simulink library "DAMA_lib"  (Simulink 6.6)
undefined symbols (not defined in the file or in its folder): aa2rot, D, DiscIntNeverNeededParam, DRprogressbar, epsilon, Kd, Ko, Kp, manip, manipulator, path_des, Q, q0, q_d0, rho, robot, show_3D, StartTime, subs, Ts, VR_handle, vrmfunc
libraries: DAMA_lib x7, vrlib x1, simulink x1
(part 2 of 4)

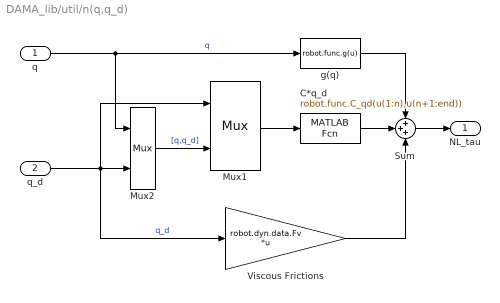
== system DAMA_lib/util/n(q,q_d) ==
  q : Inport
  q_d : Inport  Port=2
  C*q_d : MATLABFcn  MATLABFcn=robot.func.C_qd(u(1:n),u(n+1:end))  OutputDimensions=n
  Mux1 : Mux  Inputs=2
      settings: DisplayOption=signals
  Mux2 : Mux  Inputs=2
      settings: DisplayOption=signals
  Sum : Sum  Inputs=+++
  Viscous Frictions : Gain  Gain=robot.dyn.data.Fv  Multiplication=Matrix(K*u)
  g(q) : MATLABFcn  MATLABFcn=robot.func.g(u)  OutputDimensions=n
  NL_tau : Outport
  wires:
  Viscous Frictions/1 -> Sum/3
  Sum/1 -> NL_tau/1
  q/1 -> g(q)/1, Mux2/1  "q"
  q_d/1 -> Viscous Frictions/1, Mux1/1, Mux2/2  "q_d"
  C*q_d/1 -> Sum/2
  g(q)/1 -> Sum/1
  Mux2/1 -> Mux1/2  "[q,q_d]"
  Mux1/1 -> C*q_d/1

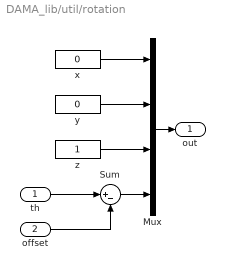
== system DAMA_lib/util/rotation ==
  th : Inport
  offset : Inport  Port=2
  Mux : Mux
  Sum : Sum  Inputs=|+-
  x : Constant  Value=0
  y : Constant  Value=0
  z : Constant
  out : Outport
  wires:
  offset/1 -> Sum/2
  Sum/1 -> Mux/4
  th/1 -> Sum/1
  Mux/1 -> out/1
  z/1 -> Mux/3
  y/1 -> Mux/2
  x/1 -> Mux/1

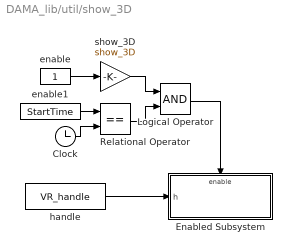
== system DAMA_lib/util/show_3D ==
  Clock : Clock
      settings: Decimation=10
  Enabled Subsystem : Subsystem  TreatAsAtomicUnit=on
  Logical Operator : Logic  AllPortsSameDT=off  OutDataTypeMode=Boolean
  Relational Operator : RelationalOperator  Operator===  LogicOutDataTypeMode=Boolean
  enable : Constant
  enable1 : Constant  Value=StartTime
  handle : Constant  Value=VR_handle
  show_3D : Gain  Gain=show_3D
  wires:
  show_3D/1 -> Logical Operator/1
  enable/1 -> show_3D/1
  handle/1 -> Enabled Subsystem/1(h)
  Logical Operator/1 -> Enabled Subsystem/Enable
  Relational Operator/1 -> Logical Operator/2
  enable1/1 -> Relational Operator/1
  Clock/1 -> Relational Operator/2

== system DAMA_lib/util/translation ==
  d : Inport
  offset : Inport  Port=2
  Mux : Mux  Inputs=3
  Sum : Sum  Inputs=|+-
  x : Constant  Value=0
  y : Constant  Value=0
  out : Outport
  wires:
  offset/1 -> Sum/2
  Sum/1 -> Mux/3
  d/1 -> Sum/1
  Mux/1 -> out/1
  y/1 -> Mux/2
  x/1 -> Mux/1

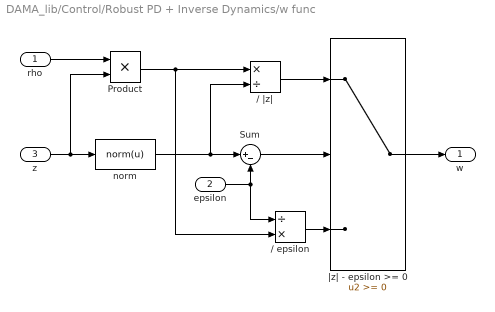
== system DAMA_lib/Control/Robust PD + Inverse Dynamics/w func ==
  rho : Inport
  epsilon : Inport  Port=2
  z : Inport  Port=3
  " / epsilon" : Product  Inputs=/*  OutScaling=2^-10
  " / |z|" : Product  Inputs=*/  OutScaling=2^-10
  Product : Product  RndMeth=Zero
  Sum : Sum  Inputs=|+-
  norm : MATLABFcn  MATLABFcn=norm(u)
  |z| - epsilon >= 0 : Switch
  w : Outport
  wires:
  z/1 -> norm/1, Product/2
  Sum/1 -> |z| - epsilon >= 0/2
  rho/1 -> Product/1
  norm/1 -> Sum/1, " / |z|"/2
  Product/1 -> " / |z|"/1, " / epsilon"/2
  " / |z|"/1 -> |z| - epsilon >= 0/1
  " / epsilon"/1 -> |z| - epsilon >= 0/3
  epsilon/1 -> Sum/2, " / epsilon"/1
  |z| - epsilon >= 0/1 -> w/1

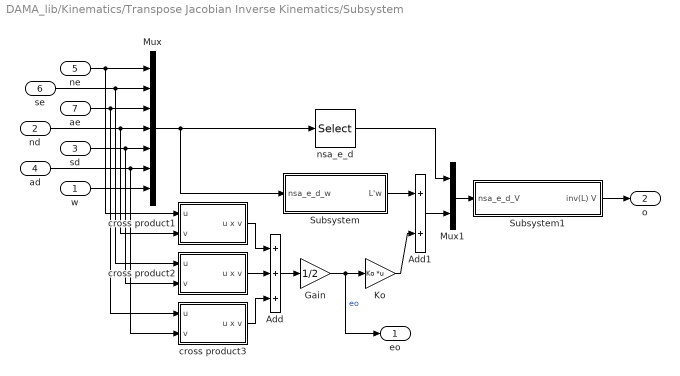
== system DAMA_lib/Kinematics/Transpose Jacobian Inverse Kinematics/Subsystem ==
  w : Inport
  nd : Inport  Port=2
  sd : Inport  Port=3
  ad : Inport  Port=4
  ne : Inport  Port=5
  se : Inport  Port=6
  ae : Inport  Port=7
  Add : Sum  Inputs=3  OutScaling=2^-10
  Add1 : Sum  Inputs=2  OutScaling=2^-10
  Gain : Gain  Gain=1/2
  Ko : Gain  Gain=Ko  Multiplication=Matrix(K*u) (u vector)
  Mux : Mux  Inputs=7
  Mux1 : Mux  Inputs=2
  Subsystem : Subsystem
  Subsystem1 : Subsystem
  cross product1 : Subsystem
  cross product2 : Subsystem
  cross product3 : Subsystem
  nsa_e_d : Selector  IndexOptions=Index vector (dialog)  Indices=[1:18]  OutputSizes=1  InputPortWidth=21
  eo : Outport
  o : Outport  Port=2
  wires:
  ne/1 -> Mux/1, cross product1/1(u)
  se/1 -> Mux/2, cross product2/1(u)
  ae/1 -> Mux/3, cross product3/1(u)
  nd/1 -> Mux/4, cross product1/2(v)
  sd/1 -> Mux/5, cross product2/2(v)
  ad/1 -> Mux/6, cross product3/2(v)
  w/1 -> Mux/7
  cross product1/1(u x v) -> Add/1
  cross product2/1(u x v) -> Add/2
  cross product3/1(u x v) -> Add/3
  Add/1 -> Gain/1
  Gain/1 -> eo/1, Ko/1  "eo"
  nsa_e_d/1 -> Mux1/1
  Mux1/1 -> Subsystem1/1(nsa_e_d_V)
  Mux/1 -> Subsystem/1(nsa_e_d_w), nsa_e_d/1
  Subsystem/1(L'w) -> Add1/1
  Ko/1 -> Add1/2
  Add1/1 -> Mux1/2
  Subsystem1/1(inv(L) V) -> o/1

== system DAMA_lib/util/show_3D/Enabled Subsystem ==
  h : Inport
  Enable : EnablePort
  show 3D : MATLABFcn  MATLABFcn=vrmfunc('FnOpen', u )  OutputDimensions=0
  wires:
  h/1 -> show 3D/1

== system DAMA_lib/Kinematics/Transpose Jacobian Inverse Kinematics/Subsystem/Subsystem ==
  nsa_e_d_w : Inport
  L'1 : Fcn  Expr=(1/2*u(12)*u(3)+1/2*u(11)*u(2)+1/2*u(15)*u(6)+1/2*u(14)*u(5)+1/2*u(18)*u(9)+1/2*u(17)*u(8))*u(19)+(-1/2*u(10)*u(2)-1/2*u(13)*u(5)-1/2*u(16)*u(8))*u(20)+(-1/2*u(10)*u(3)-1/2*u(13)*u(6)-1/2*u(16)*u(9))*u(21)
  L'2 : Fcn  Expr=(-1/2*u(11)*u(1)-1/2*u(14)*u(4)-1/2*u(17)*u(7))*u(19)+(1/2*u(12)*u(3)+1/2*u(10)*u(1)+1/2*u(15)*u(6)+1/2*u(13)*u(4)+1/2*u(18)*u(9)+1/2*u(16)*u(7))*u(20)+(-1/2*u(11)*u(3)-1/2*u(14)*u(6)-1/2*u(17)*u(9))*u(21)
  L'3 : Fcn  Expr=(-1/2*u(12)*u(1)-1/2*u(15)*u(4)-1/2*u(18)*u(7))*u(19)+(-1/2*u(12)*u(2)-1/2*u(15)*u(5)-1/2*u(18)*u(8))*u(20)+(1/2*u(11)*u(2)+1/2*u(10)*u(1)+1/2*u(14)*u(5)+1/2*u(13)*u(4)+1/2*u(17)*u(8)+1/2*u(16)*u(7))*u(21)
  Mux : Mux  Inputs=3
  L'w : Outport
  wires:
  nsa_e_d_w/1 -> L'1/1, L'2/1, L'3/1
  L'1/1 -> Mux/1
  L'2/1 -> Mux/2
  L'3/1 -> Mux/3
  Mux/1 -> L'w/1
